simulink model "lunar_lander_sim_MPC"  (R2023a)
settings: Solver=VariableStepAuto  StartTime=0.0  StopTime=10.0  RelTol=1e-3
undefined symbols (not defined in the file or in its folder): A, aMode
libraries: simulink_extras x7, mpclib x2, shared6dofsys x2, sharedutil x2
settings Model: Creator=cnsl  LastModifiedBy=cnsl

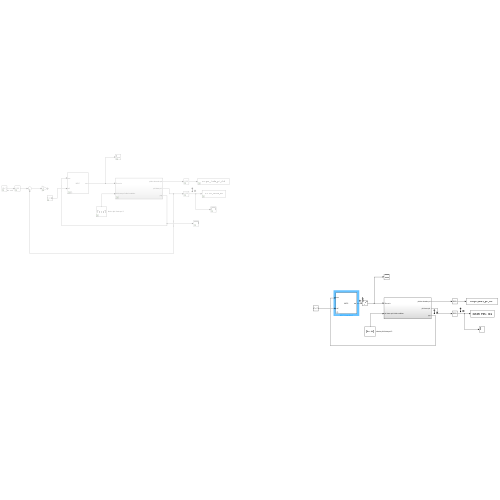
[thumbnail: Simulink's stored preview of the top-level diagram]
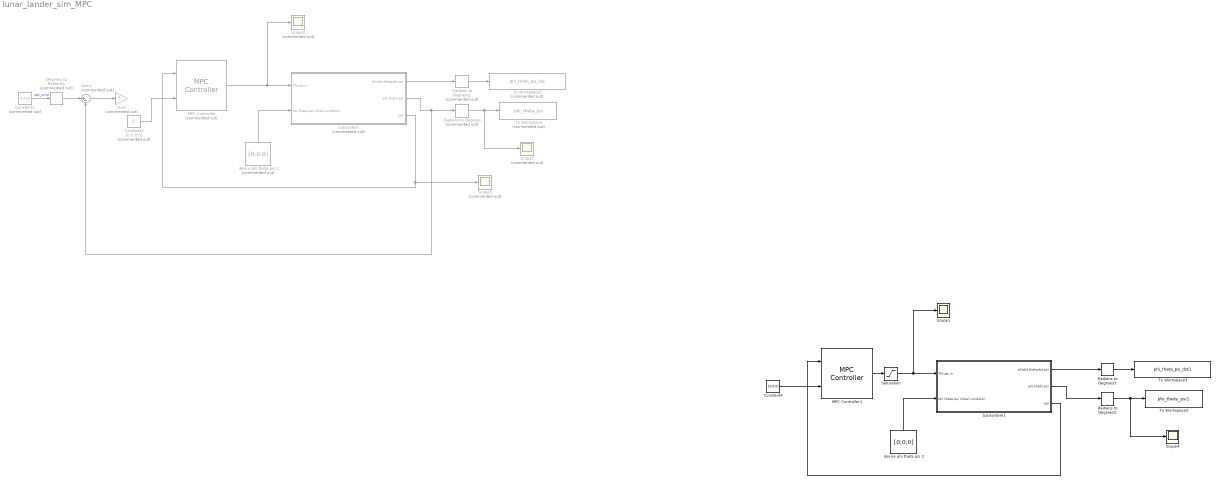
== system lunar_lander_sim_MPC ==
  Constant1 : Constant  Commented=on  Value=[5;0;0]
  Constant2 : Constant  Commented=on  Value=[0.5;0;0]
  Constant4 : Constant  Value=[0;0;0]
  Degrees to Radians1 : simulink_extras/Transformations/Degrees to Radians  Commented=on
  Gain : Gain  Commented=on  Gain=5
  MPC Controller : mpclib/MPC Controller  Commented=on  SCDEnableBlockLinearizationSpecification=on  mpcobj=mpc_stabilization_LL  is_multiple=0  enable_value=0  return_u0=off  updateMPCinCallerWorkspace=on  md_inport=off  mv_inport=off  uref_inport=off  return_cost=off  return_mvseq=off  return_qpstatus=off  return_xseq=off  return_state=off  return_ovseq=off  state_inport=off  umin_inport=off  umax_inport=off  ymin_inport=off  ymax_inport=off  cc_inport=off  ywt_inport=off  uwt_inport=off  duwt_inport=off  rhoeps_inport=off  pm_inport=off  MaximumP=10  HorizonChoice=FixedHorizon  n_ts=0.01  n_p=10  n_mv=8  n_md=0  n_ud=0  n_mo=3  n_uo=0  BlockDataType=double  SampleTimeInherited=off  switch_inport=off
  MPC Controller1 : mpclib/MPC Controller  SCDEnableBlockLinearizationSpecification=on  is_multiple=0  enable_value=0  return_u0=off  updateMPCinCallerWorkspace=on  md_inport=off  mv_inport=off  uref_inport=off  return_cost=off  return_mvseq=off  return_qpstatus=off  return_xseq=off  return_state=off  return_ovseq=off  state_inport=off  umin_inport=off  umax_inport=off  ymin_inport=off  ymax_inport=off  cc_inport=off  ywt_inport=off  uwt_inport=off  duwt_inport=off  rhoeps_inport=off  pm_inport=off  MaximumP=10  HorizonChoice=FixedHorizon  n_ts=0.1  n_p=10  n_mv=8  n_md=1  n_ud=0  n_mo=3  n_uo=0  BlockDataType=double  SampleTimeInherited=off  switch_inport=off
  Radians to Degrees : simulink_extras/Transformations/Radians to Degrees  Commented=on
  Radians to Degrees1 : simulink_extras/Transformations/Radians to Degrees  Commented=on
  Radians to Degrees2 : simulink_extras/Transformations/Radians to Degrees
  Radians to Degrees3 : simulink_extras/Transformations/Radians to Degrees
  Saturation : Saturate  UpperLimit=10  LowerLimit=0
  Scope1 : Scope
  Scope2 : Scope  Commented=on
  Scope3 : Scope  Commented=on
  Scope4 : Scope
  Scope5 : Scope  Commented=on
  Subsystem : Subsystem  Commented=on
  Subsystem1 : Subsystem
  Sum1 : Sum  Commented=on  Inputs=|+-
  To Workspace : ToWorkspace  Commented=on  VariableName=phi_theta_psi  SaveFormat=Timeseries  SampleTime=-1
  To Workspace1 : ToWorkspace  Commented=on  VariableName=phi_theta_psi_dot  SaveFormat=Timeseries  SampleTime=-1
  To Workspace2 : ToWorkspace  VariableName=phi_theta_psi1  SaveFormat=Timeseries  SampleTime=-1
  To Workspace3 : ToWorkspace  VariableName=phi_theta_psi_dot1  SaveFormat=Timeseries  SampleTime=-1
  desire phi theta psi 1 : Constant  Commented=on  Value=[0;0;0]
  desire phi theta psi 2 : Constant  Value=[0;0;0]
  wires:
  Subsystem/2("phi theta psi ") -> Radians to Degrees/1, Sum1/2
  Subsystem/1(phidot thetadot psi) -> Radians to Degrees1/1
  Radians to Degrees/1 -> Scope3/1, To Workspace/1
  desire phi theta psi 1/1 -> Subsystem/2("phi theta psi initial condition ")
  Radians to Degrees1/1 -> To Workspace1/1
  MPC Controller/1 -> Scope2/1, Subsystem/1(Thrust in)
  Subsystem/3(" pqr") -> Scope5/1, MPC Controller/1
  Constant1/1 -> Degrees to Radians1/1  "pqr_cmd"
  Degrees to Radians1/1 -> Sum1/1
  Sum1/1 -> Gain/1
  Constant2/1 -> MPC Controller/2
  Radians to Degrees2/1 -> Scope4/1, To Workspace2/1
  Subsystem1/2("phi theta psi ") -> Radians to Degrees2/1
  desire phi theta psi 2/1 -> Subsystem1/2("phi theta psi initial condition ")
  Radians to Degrees3/1 -> To Workspace3/1
  Constant4/1 -> MPC Controller1/2
  MPC Controller1/1 -> Saturation/1
  Subsystem1/1(phidot thetadot psi) -> Radians to Degrees3/1
  Subsystem1/3(" pqr") -> MPC Controller1/1
  Saturation/1 -> Scope1/1, Subsystem1/1(Thrust in)

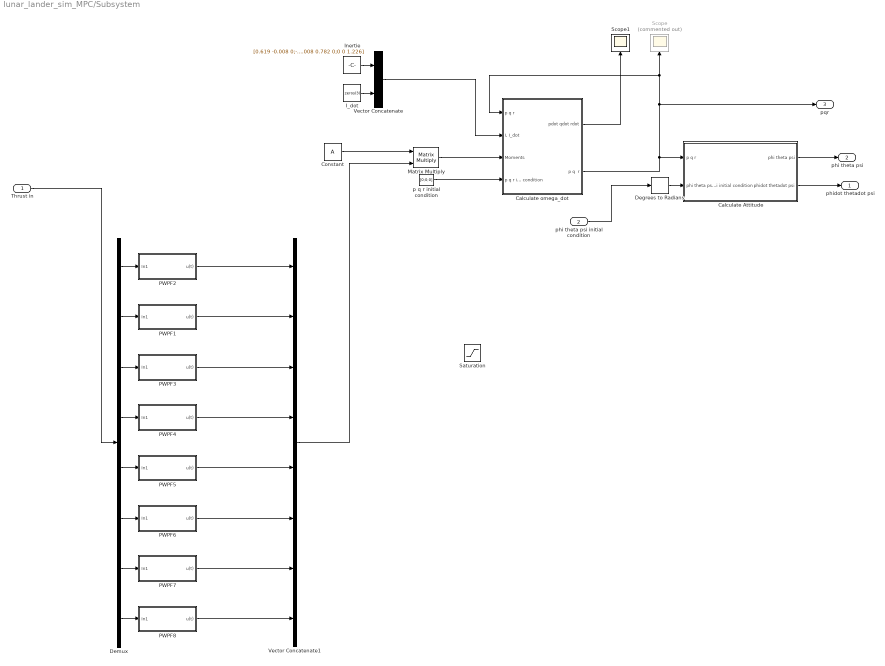
== system lunar_lander_sim_MPC/Subsystem ==
  Thrust in : Inport
  "phi theta psi initial condition " : Inport  Port=2
  " p q r initial condition" : Constant  Value=[0;0;0]
  "Calculate Attitude " : Subsystem
  Calculate omega_dot : Subsystem  AncestorBlock=shared6dofsys/Calculate omega_dot  mask{aMode=aMode}
      mask init:
      | if aerosharedtest(gcb)
      |     aerosharedicon('shared');
      | else
      |     sharedautoicon('shared');
      | end
      settings: LibrarySourceBlock=shared6dofsys/Calculate omega_dot
  Constant : Constant  Value=A
  Degrees to Radians : simulink_extras/Transformations/Degrees to Radians
  Demux : Demux  Outputs=8
  I_dot : Constant  Value=zeros(3)
  Inertie : Constant  Value=[0.619 -0.008 0;-0.008 0.782 0;0 0 1.226]
  Matrix Multiply : Product  Multiplication=Matrix(*)
  PWPF1 : Subsystem
  PWPF2 : Subsystem
  PWPF3 : Subsystem
  PWPF4 : Subsystem
  PWPF5 : Subsystem
  PWPF6 : Subsystem
  PWPF7 : Subsystem
  PWPF8 : Subsystem
  Saturation : Saturate
  Scope : Scope  Commented=on
  Scope1 : Scope
  Vector Concatenate : Concatenate  Mode=Multidimensional array
  Vector Concatenate1 : Concatenate  NumInputs=8
  phidot thetadot psi : Outport
  "phi theta psi " : Outport  Port=2
  " pqr" : Outport  Port=3
  wires:
  Vector Concatenate/1 -> Calculate omega_dot/2("I, I_dot")
  Inertie/1 -> Vector Concatenate/1
  Calculate omega_dot/2(p q  r) -> Scope/1, Calculate omega_dot/1(p q r), " pqr"/1, "Calculate Attitude "/1(p q r)
  I_dot/1 -> Vector Concatenate/2
  " p q r initial condition"/1 -> Calculate omega_dot/4(p q r initial condition)
  "Calculate Attitude "/1("phi theta psi ") -> "phi theta psi "/1
  Degrees to Radians/1 -> "Calculate Attitude "/2("phi theta psi initial condition ")
  "phi theta psi initial condition "/1 -> Degrees to Radians/1
  "Calculate Attitude "/2(phidot thetadot psi) -> phidot thetadot psi/1
  Calculate omega_dot/1(pdot qdot rdot) -> Scope1/1
  Matrix Multiply/1 -> Calculate omega_dot/3(Moments)
  Constant/1 -> Matrix Multiply/1
  Thrust in/1 -> Demux/1
  Demux/1 -> PWPF2/1(In1)
  Demux/2 -> PWPF1/1(In1)
  Demux/3 -> PWPF3/1(In1)
  Demux/4 -> PWPF4/1(In1)
  Demux/5 -> PWPF5/1(In1)
  Demux/6 -> PWPF6/1(In1)
  Demux/7 -> PWPF7/1(In1)
  Demux/8 -> PWPF8/1(In1)
  PWPF2/1(u(t)) -> Vector Concatenate1/1
  PWPF1/1(u(t)) -> Vector Concatenate1/2
  PWPF3/1(u(t)) -> Vector Concatenate1/3
  PWPF4/1(u(t)) -> Vector Concatenate1/4
  PWPF5/1(u(t)) -> Vector Concatenate1/5
  PWPF6/1(u(t)) -> Vector Concatenate1/6
  PWPF7/1(u(t)) -> Vector Concatenate1/7
  Vector Concatenate1/1 -> Matrix Multiply/2
  PWPF8/1(u(t)) -> Vector Concatenate1/8

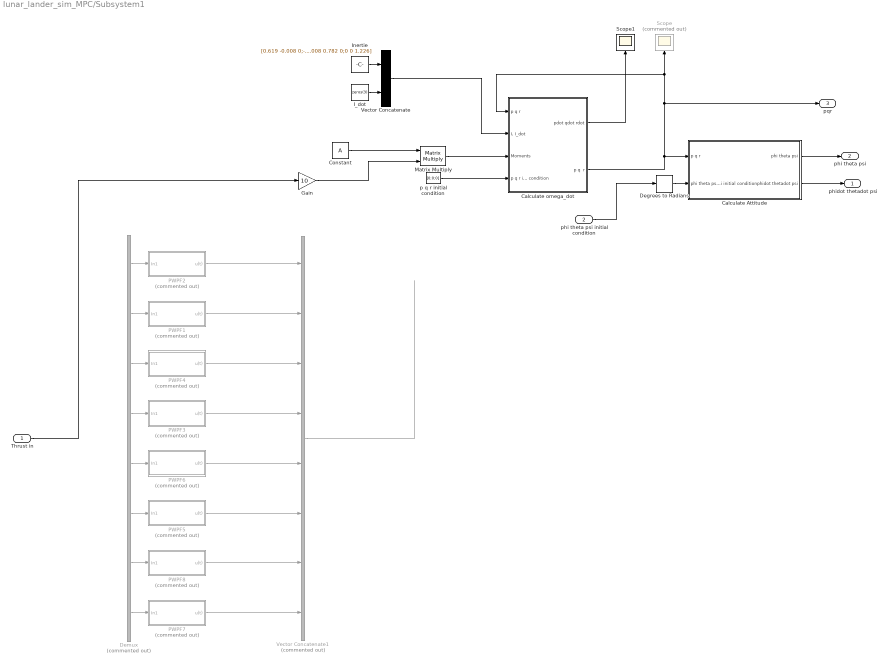
== system lunar_lander_sim_MPC/Subsystem1 ==
  Thrust in : Inport
  "phi theta psi initial condition " : Inport  Port=2
  " p q r initial condition" : Constant  Value=[0;0;0]
  "Calculate Attitude " : Subsystem
  Calculate omega_dot : Subsystem  AncestorBlock=shared6dofsys/Calculate omega_dot  mask{aMode=aMode}
      mask init:
      | if aerosharedtest(gcb)
      |     aerosharedicon('shared');
      | else
      |     sharedautoicon('shared');
      | end
      settings: LibrarySourceBlock=shared6dofsys/Calculate omega_dot
  Constant : Constant  Value=A
  Degrees to Radians : simulink_extras/Transformations/Degrees to Radians
  Demux : Demux  Commented=on  Outputs=8
  Gain : Gain  Gain=10
  I_dot : Constant  Value=zeros(3)
  Inertie : Constant  Value=[0.619 -0.008 0;-0.008 0.782 0;0 0 1.226]
  Matrix Multiply : Product  Multiplication=Matrix(*)
  PWPF1 : Subsystem  Commented=on
  PWPF2 : Subsystem  Commented=on
  PWPF3 : Subsystem  Commented=on
  PWPF4 : Subsystem  Commented=on
  PWPF5 : Subsystem  Commented=on
  PWPF6 : Subsystem  Commented=on
  PWPF7 : Subsystem  Commented=on
  PWPF8 : Subsystem  Commented=on
  Scope : Scope  Commented=on
  Scope1 : Scope
  Vector Concatenate : Concatenate  Mode=Multidimensional array
  Vector Concatenate1 : Concatenate  Commented=on  NumInputs=8
  phidot thetadot psi : Outport
  "phi theta psi " : Outport  Port=2
  " pqr" : Outport  Port=3
  wires:
  Vector Concatenate/1 -> Calculate omega_dot/2("I, I_dot")
  Inertie/1 -> Vector Concatenate/1
  Calculate omega_dot/2(p q  r) -> Scope/1, Calculate omega_dot/1(p q r), " pqr"/1, "Calculate Attitude "/1(p q r)
  I_dot/1 -> Vector Concatenate/2
  " p q r initial condition"/1 -> Calculate omega_dot/4(p q r initial condition)
  "Calculate Attitude "/1("phi theta psi ") -> "phi theta psi "/1
  Degrees to Radians/1 -> "Calculate Attitude "/2("phi theta psi initial condition ")
  "phi theta psi initial condition "/1 -> Degrees to Radians/1
  "Calculate Attitude "/2(phidot thetadot psi) -> phidot thetadot psi/1
  Calculate omega_dot/1(pdot qdot rdot) -> Scope1/1
  Matrix Multiply/1 -> Calculate omega_dot/3(Moments)
  Constant/1 -> Matrix Multiply/1
  Thrust in/1 -> Gain/1
  Demux/1 -> PWPF2/1(In1)
  Demux/2 -> PWPF1/1(In1)
  Demux/3 -> PWPF4/1(In1)
  Demux/4 -> PWPF3/1(In1)
  Demux/5 -> PWPF6/1(In1)
  Demux/6 -> PWPF5/1(In1)
  Demux/7 -> PWPF8/1(In1)
  Demux/8 -> PWPF7/1(In1)
  PWPF2/1(u(t)) -> Vector Concatenate1/1
  PWPF1/1(u(t)) -> Vector Concatenate1/2
  PWPF4/1(u(t)) -> Vector Concatenate1/3
  PWPF3/1(u(t)) -> Vector Concatenate1/4
  PWPF6/1(u(t)) -> Vector Concatenate1/5
  PWPF5/1(u(t)) -> Vector Concatenate1/6
  PWPF8/1(u(t)) -> Vector Concatenate1/7
  Vector Concatenate1/1 -> ?
  PWPF7/1(u(t)) -> Vector Concatenate1/8
  Gain/1 -> Matrix Multiply/2

== system lunar_lander_sim_MPC/Subsystem/Calculate Attitude  ==
  p q r : Inport
  "phi theta psi initial condition " : Inport  Port=2
  " " : Integrator  InitialConditionSource=external
  phidot thetadot psidot : shared6dofsys/DCM & Euler Angles (Euler)/phidot thetadot psidot  SystemSampleTime=-1  VariantActivationTime=update diagram  Latency=0  AutoFrameSizeCalculation=off
  "phi theta psi " : Outport
  phidot thetadot psi : Outport  Port=2
  wires:
  "phi theta psi initial condition "/1 -> " "/2
  " "/1 -> phidot thetadot psidot/2, "phi theta psi "/1
  phidot thetadot psidot/1 -> phidot thetadot psi/1, " "/1
  p q r/1 -> phidot thetadot psidot/1

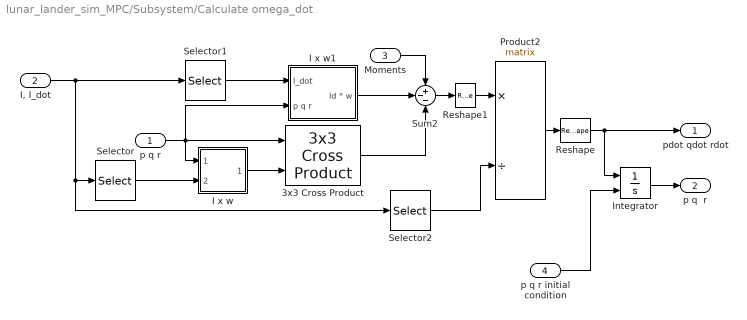
== system lunar_lander_sim_MPC/Subsystem/Calculate omega_dot ==
  p q r : Inport  OutDataTypeStr=double
  "I, I_dot" : Inport  Port=2  OutDataTypeStr=double
  Moments : Inport  Port=3  OutDataTypeStr=double
  p q r initial condition : Inport  Port=4
  3x3 Cross Product : sharedutil/3x3 Cross Product  aMode=aMode
  I x w : Subsystem
  I x w1 : Subsystem
  Integrator : Integrator  InitialConditionSource=external
  Product2 : Product  Inputs=*/  Multiplication=Matrix(*)  SaturateOnIntegerOverflow=on  OutDataTypeStr=Inherit: Same as first input
  Reshape : Reshape
  Reshape1 : Reshape  OutputDimensionality=Row vector (2-D)
  Selector : Selector  NumberOfDimensions=2  InputPortWidth=2  IndexOptions=Index vector (dialog),Select all  Indices=1:3,-1  OutputSizes=1
  Selector1 : Selector  NumberOfDimensions=2  InputPortWidth=2  IndexOptions=Index vector (dialog),Select all  Indices=4:6,-1  OutputSizes=1
  Selector2 : Selector  NumberOfDimensions=2  InputPortWidth=2  IndexOptions=Index vector (dialog),Select all  Indices=1:3,-1  OutputSizes=1
  Sum2 : Sum  Inputs=+--  SaturateOnIntegerOverflow=on
  pdot qdot rdot : Outport  OutDataTypeStr=double  VectorParamsAs1DForOutWhenUnconnected=off
  p q  r : Outport  Port=2
  wires:
  p q r initial condition/1 -> Integrator/2
  Integrator/1 -> p q  r/1
  Reshape/1 -> pdot qdot rdot/1, Integrator/1
  Selector/1 -> I x w/2(Inertia)
  Selector2/1 -> Product2/2
  "I, I_dot"/1 -> Selector/1, Selector2/1, Selector1/1
  p q r/1 -> 3x3 Cross Product/1, I x w1/2(p q r), I x w/1(p q r)
  Product2/1 -> Reshape/1
  Sum2/1 -> Reshape1/1
  Moments/1 -> Sum2/1
  I x w1/1(Id * w) -> Sum2/2
  Selector1/1 -> I x w1/1(I_dot)
  I x w/1(I * w) -> 3x3 Cross Product/2
  Reshape1/1 -> Product2/1
  3x3 Cross Product/1 -> Sum2/3

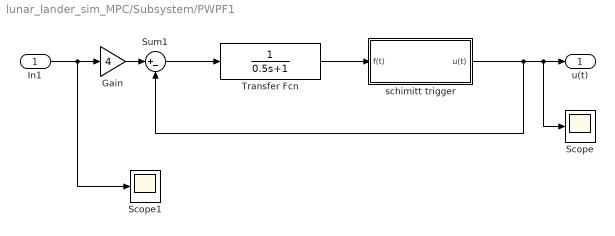
== system lunar_lander_sim_MPC/Subsystem/PWPF1 ==
  In1 : Inport
  Gain : Gain  Gain=4
  Scope : Scope
  Scope1 : Scope
  Sum1 : Sum  Inputs=|+-
  Transfer Fcn : TransferFcn  Denominator=[0.5 1]
  schimitt trigger : Subsystem
  u(t) : Outport
  wires:
  In1/1 -> Gain/1, Scope1/1
  Transfer Fcn/1 -> schimitt trigger/1(f(t))
  Sum1/1 -> Transfer Fcn/1
  Gain/1 -> Sum1/1
  schimitt trigger/1(u(t)) -> Sum1/2, u(t)/1, Scope/1

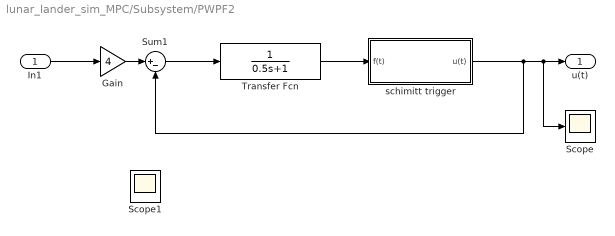
== system lunar_lander_sim_MPC/Subsystem/PWPF2 ==
  In1 : Inport
  Gain : Gain  Gain=4
  Scope : Scope
  Scope1 : Scope
  Sum1 : Sum  Inputs=|+-
  Transfer Fcn : TransferFcn  Denominator=[0.5 1]
  schimitt trigger : Subsystem
  u(t) : Outport
  wires:
  schimitt trigger/1(u(t)) -> Scope/1, u(t)/1, Sum1/2
  Gain/1 -> Sum1/1
  Sum1/1 -> Transfer Fcn/1
  Transfer Fcn/1 -> schimitt trigger/1(f(t))
  In1/1 -> Gain/1

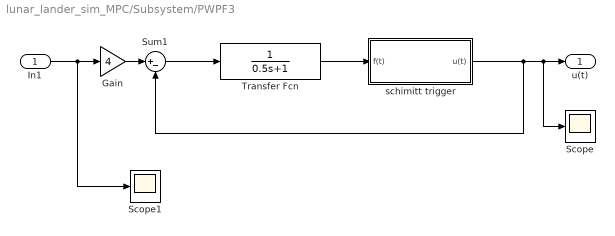
== system lunar_lander_sim_MPC/Subsystem/PWPF3 ==
  In1 : Inport
  Gain : Gain  Gain=4
  Scope : Scope
  Scope1 : Scope
  Sum1 : Sum  Inputs=|+-
  Transfer Fcn : TransferFcn  Denominator=[0.5 1]
  schimitt trigger : Subsystem
  u(t) : Outport
  wires:
  schimitt trigger/1(u(t)) -> Scope/1, u(t)/1, Sum1/2
  Gain/1 -> Sum1/1
  Sum1/1 -> Transfer Fcn/1
  Transfer Fcn/1 -> schimitt trigger/1(f(t))
  In1/1 -> Scope1/1, Gain/1

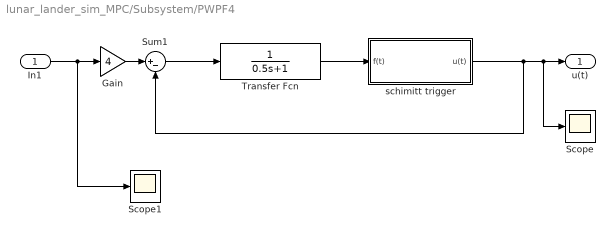
== system lunar_lander_sim_MPC/Subsystem/PWPF4 ==
  In1 : Inport
  Gain : Gain  Gain=4
  Scope : Scope
  Scope1 : Scope
  Sum1 : Sum  Inputs=|+-
  Transfer Fcn : TransferFcn  Denominator=[0.5 1]
  schimitt trigger : Subsystem
  u(t) : Outport
  wires:
  In1/1 -> Gain/1, Scope1/1
  Transfer Fcn/1 -> schimitt trigger/1(f(t))
  Sum1/1 -> Transfer Fcn/1
  Gain/1 -> Sum1/1
  schimitt trigger/1(u(t)) -> Sum1/2, u(t)/1, Scope/1

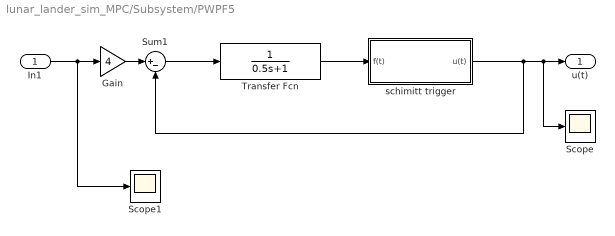
== system lunar_lander_sim_MPC/Subsystem/PWPF5 ==
  In1 : Inport
  Gain : Gain  Gain=4
  Scope : Scope
  Scope1 : Scope
  Sum1 : Sum  Inputs=|+-
  Transfer Fcn : TransferFcn  Denominator=[0.5 1]
  schimitt trigger : Subsystem
  u(t) : Outport
  wires:
  schimitt trigger/1(u(t)) -> Scope/1, u(t)/1, Sum1/2
  Gain/1 -> Sum1/1
  Sum1/1 -> Transfer Fcn/1
  Transfer Fcn/1 -> schimitt trigger/1(f(t))
  In1/1 -> Scope1/1, Gain/1

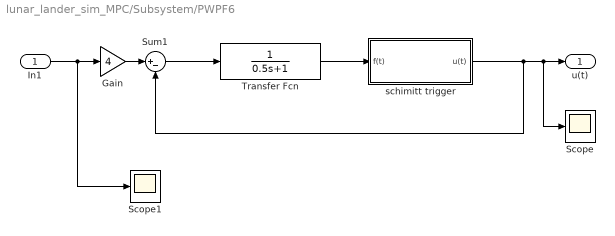
== system lunar_lander_sim_MPC/Subsystem/PWPF6 ==
  In1 : Inport
  Gain : Gain  Gain=4
  Scope : Scope
  Scope1 : Scope
  Sum1 : Sum  Inputs=|+-
  Transfer Fcn : TransferFcn  Denominator=[0.5 1]
  schimitt trigger : Subsystem
  u(t) : Outport
  wires:
  In1/1 -> Gain/1, Scope1/1
  Transfer Fcn/1 -> schimitt trigger/1(f(t))
  Sum1/1 -> Transfer Fcn/1
  Gain/1 -> Sum1/1
  schimitt trigger/1(u(t)) -> Sum1/2, u(t)/1, Scope/1

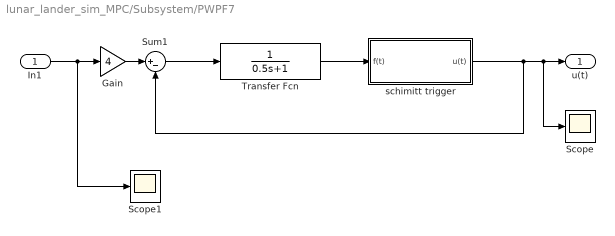
== system lunar_lander_sim_MPC/Subsystem/PWPF7 ==
  In1 : Inport
  Gain : Gain  Gain=4
  Scope : Scope
  Scope1 : Scope
  Sum1 : Sum  Inputs=|+-
  Transfer Fcn : TransferFcn  Denominator=[0.5 1]
  schimitt trigger : Subsystem
  u(t) : Outport
  wires:
  schimitt trigger/1(u(t)) -> Scope/1, u(t)/1, Sum1/2
  Gain/1 -> Sum1/1
  Sum1/1 -> Transfer Fcn/1
  Transfer Fcn/1 -> schimitt trigger/1(f(t))
  In1/1 -> Scope1/1, Gain/1

== system lunar_lander_sim_MPC/Subsystem/PWPF8 ==
  In1 : Inport
  Gain : Gain  Gain=4
  Scope : Scope
  Scope1 : Scope
  Sum1 : Sum  Inputs=|+-
  Transfer Fcn : TransferFcn  Denominator=[0.5 1]
  schimitt trigger : Subsystem
  u(t) : Outport
  wires:
  In1/1 -> Gain/1, Scope1/1
  Transfer Fcn/1 -> schimitt trigger/1(f(t))
  Sum1/1 -> Transfer Fcn/1
  Gain/1 -> Sum1/1
  schimitt trigger/1(u(t)) -> Sum1/2, u(t)/1, Scope/1

== system lunar_lander_sim_MPC/Subsystem1/Calculate Attitude  ==
  p q r : Inport
  "phi theta psi initial condition " : Inport  Port=2
  " " : Integrator  InitialConditionSource=external
  phidot thetadot psidot : shared6dofsys/DCM & Euler Angles (Euler)/phidot thetadot psidot  SystemSampleTime=-1  VariantActivationTime=update diagram  Latency=0  AutoFrameSizeCalculation=off
  "phi theta psi " : Outport
  phidot thetadot psi : Outport  Port=2
  wires:
  "phi theta psi initial condition "/1 -> " "/2
  " "/1 -> phidot thetadot psidot/2, "phi theta psi "/1
  phidot thetadot psidot/1 -> phidot thetadot psi/1, " "/1
  p q r/1 -> phidot thetadot psidot/1

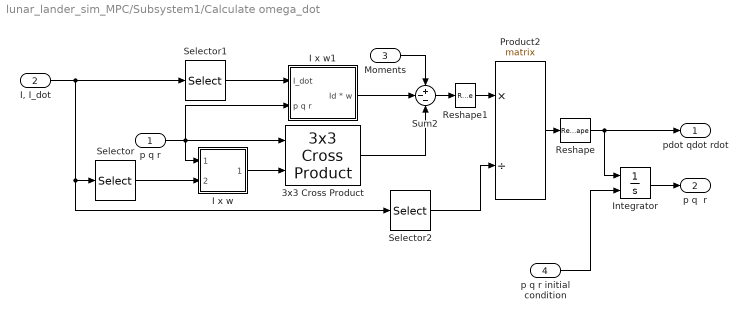
== system lunar_lander_sim_MPC/Subsystem1/Calculate omega_dot ==
  p q r : Inport  OutDataTypeStr=double
  "I, I_dot" : Inport  Port=2  OutDataTypeStr=double
  Moments : Inport  Port=3  OutDataTypeStr=double
  p q r initial condition : Inport  Port=4
  3x3 Cross Product : sharedutil/3x3 Cross Product  aMode=aMode
  I x w : Subsystem
  I x w1 : Subsystem
  Integrator : Integrator  InitialConditionSource=external
  Product2 : Product  Inputs=*/  Multiplication=Matrix(*)  SaturateOnIntegerOverflow=on  OutDataTypeStr=Inherit: Same as first input
  Reshape : Reshape
  Reshape1 : Reshape  OutputDimensionality=Row vector (2-D)
  Selector : Selector  NumberOfDimensions=2  InputPortWidth=2  IndexOptions=Index vector (dialog),Select all  Indices=1:3,-1  OutputSizes=1
  Selector1 : Selector  NumberOfDimensions=2  InputPortWidth=2  IndexOptions=Index vector (dialog),Select all  Indices=4:6,-1  OutputSizes=1
  Selector2 : Selector  NumberOfDimensions=2  InputPortWidth=2  IndexOptions=Index vector (dialog),Select all  Indices=1:3,-1  OutputSizes=1
  Sum2 : Sum  Inputs=+--  SaturateOnIntegerOverflow=on
  pdot qdot rdot : Outport  OutDataTypeStr=double  VectorParamsAs1DForOutWhenUnconnected=off
  p q  r : Outport  Port=2
  wires:
  p q r initial condition/1 -> Integrator/2
  Integrator/1 -> p q  r/1
  Reshape/1 -> pdot qdot rdot/1, Integrator/1
  Selector/1 -> I x w/2(Inertia)
  Selector2/1 -> Product2/2
  "I, I_dot"/1 -> Selector/1, Selector2/1, Selector1/1
  p q r/1 -> 3x3 Cross Product/1, I x w1/2(p q r), I x w/1(p q r)
  Product2/1 -> Reshape/1
  Sum2/1 -> Reshape1/1
  Moments/1 -> Sum2/1
  I x w1/1(Id * w) -> Sum2/2
  Selector1/1 -> I x w1/1(I_dot)
  I x w/1(I * w) -> 3x3 Cross Product/2
  Reshape1/1 -> Product2/1
  3x3 Cross Product/1 -> Sum2/3

== system lunar_lander_sim_MPC/Subsystem1/PWPF1 ==
  In1 : Inport
  Gain : Gain  Gain=4
  Scope : Scope
  Scope1 : Scope
  schimitt trigger : Subsystem
  u(t) : Outport
  wires:
  In1/1 -> Gain/1, Scope1/1
  Gain/1 -> schimitt trigger/1(f(t))
  schimitt trigger/1(u(t)) -> u(t)/1, Scope/1

== system lunar_lander_sim_MPC/Subsystem1/PWPF2 ==
  In1 : Inport
  Gain : Gain  Gain=4
  Scope : Scope
  Scope1 : Scope
  schimitt trigger : Subsystem
  u(t) : Outport
  wires:
  schimitt trigger/1(u(t)) -> Scope/1, u(t)/1
  Gain/1 -> schimitt trigger/1(f(t))
  In1/1 -> Scope1/1, Gain/1

== system lunar_lander_sim_MPC/Subsystem1/PWPF3 ==
  In1 : Inport
  Gain : Gain  Gain=4
  Scope : Scope
  Scope1 : Scope
  schimitt trigger : Subsystem
  u(t) : Outport
  wires:
  schimitt trigger/1(u(t)) -> Scope/1, u(t)/1
  Gain/1 -> schimitt trigger/1(f(t))
  In1/1 -> Scope1/1, Gain/1

== system lunar_lander_sim_MPC/Subsystem1/PWPF4 ==
  In1 : Inport
  Gain : Gain  Gain=4
  Scope : Scope
  Scope1 : Scope
  schimitt trigger : Subsystem
  u(t) : Outport
  wires:
  In1/1 -> Gain/1, Scope1/1
  Gain/1 -> schimitt trigger/1(f(t))
  schimitt trigger/1(u(t)) -> u(t)/1, Scope/1

== system lunar_lander_sim_MPC/Subsystem1/PWPF5 ==
  In1 : Inport
  Gain : Gain  Gain=4
  Scope : Scope
  Scope1 : Scope
  schimitt trigger : Subsystem
  u(t) : Outport
  wires:
  schimitt trigger/1(u(t)) -> Scope/1, u(t)/1
  Gain/1 -> schimitt trigger/1(f(t))
  In1/1 -> Scope1/1, Gain/1

== system lunar_lander_sim_MPC/Subsystem1/PWPF6 ==
  In1 : Inport
  Gain : Gain  Gain=4
  Scope : Scope
  Scope1 : Scope
  schimitt trigger : Subsystem
  u(t) : Outport
  wires:
  In1/1 -> Gain/1, Scope1/1
  Gain/1 -> schimitt trigger/1(f(t))
  schimitt trigger/1(u(t)) -> u(t)/1, Scope/1

== system lunar_lander_sim_MPC/Subsystem1/PWPF7 ==
  In1 : Inport
  Gain : Gain  Gain=4
  Scope : Scope
  Scope1 : Scope
  schimitt trigger : Subsystem
  u(t) : Outport
  wires:
  In1/1 -> Gain/1, Scope1/1
  Gain/1 -> schimitt trigger/1(f(t))
  schimitt trigger/1(u(t)) -> u(t)/1, Scope/1

== system lunar_lander_sim_MPC/Subsystem1/PWPF8 ==
  In1 : Inport
  Gain : Gain  Gain=4
  Scope : Scope
  Scope1 : Scope
  schimitt trigger : Subsystem
  u(t) : Outport
  wires:
  schimitt trigger/1(u(t)) -> Scope/1, u(t)/1
  Gain/1 -> schimitt trigger/1(f(t))
  In1/1 -> Scope1/1, Gain/1

== system lunar_lander_sim_MPC/Subsystem/Calculate omega_dot/I x w ==
  p q r : Inport
  Inertia : Inport  Port=2
  Product : Product  Multiplication=Matrix(*)  InputSameDT=on  SaturateOnIntegerOverflow=on  OutDataTypeStr=Inherit: Same as first input
  Reshape1 : Reshape  OutputDimensionality=Column vector (2-D)
  Reshape2 : Reshape
  I * w : Outport  VectorParamsAs1DForOutWhenUnconnected=off
  wires:
  Product/1 -> Reshape2/1
  Inertia/1 -> Product/1
  p q r/1 -> Reshape1/1
  Reshape1/1 -> Product/2
  Reshape2/1 -> I * w/1

== system lunar_lander_sim_MPC/Subsystem/Calculate omega_dot/I x w1 ==
  I_dot : Inport
  p q r : Inport  Port=2
  Product : Product  Multiplication=Matrix(*)  InputSameDT=on  SaturateOnIntegerOverflow=on  OutDataTypeStr=Inherit: Same as first input
  Reshape1 : Reshape  OutputDimensionality=Column vector (2-D)
  Reshape2 : Reshape
  Id * w : Outport  VectorParamsAs1DForOutWhenUnconnected=off
  wires:
  p q r/1 -> Reshape1/1
  I_dot/1 -> Product/1
  Product/1 -> Reshape2/1
  Reshape1/1 -> Product/2
  Reshape2/1 -> Id * w/1

== system lunar_lander_sim_MPC/Subsystem/PWPF1/schimitt trigger ==
  f(t) : Inport
  Gain : Gain  Gain=-1
  Relay : Relay  OnSwitchValue=0.45  OffSwitchValue=0.15  OnOutputValue=10
  Relay1 : Relay  OnSwitchValue=0.45  OffSwitchValue=0.15  OnOutputValue=-10
  Switch : Switch  Criteria=u2 > Threshold  SaturateOnIntegerOverflow=off  InputSameDT=off
  u(t) : Outport
  wires:
  Switch/1 -> u(t)/1
  Relay/1 -> Switch/1
  Gain/1 -> Relay1/1
  Relay1/1 -> Switch/3
  f(t)/1 -> Switch/2, Gain/1, Relay/1

== system lunar_lander_sim_MPC/Subsystem/PWPF2/schimitt trigger ==
  f(t) : Inport
  Gain : Gain  Gain=-1
  Relay : Relay  OnSwitchValue=0.45  OffSwitchValue=0.15  OnOutputValue=10
  Relay1 : Relay  OnSwitchValue=0.45  OffSwitchValue=0.15  OnOutputValue=-10
  Switch : Switch  Criteria=u2 > Threshold  SaturateOnIntegerOverflow=off  InputSameDT=off
  u(t) : Outport
  wires:
  f(t)/1 -> Relay/1, Gain/1, Switch/2
  Relay1/1 -> Switch/3
  Gain/1 -> Relay1/1
  Relay/1 -> Switch/1
  Switch/1 -> u(t)/1

== system lunar_lander_sim_MPC/Subsystem/PWPF3/schimitt trigger ==
  f(t) : Inport
  Gain : Gain  Gain=-1
  Relay : Relay  OnSwitchValue=0.45  OffSwitchValue=0.15  OnOutputValue=10
  Relay1 : Relay  OnSwitchValue=0.45  OffSwitchValue=0.15  OnOutputValue=-10
  Switch : Switch  Criteria=u2 > Threshold  SaturateOnIntegerOverflow=off  InputSameDT=off
  u(t) : Outport
  wires:
  f(t)/1 -> Relay/1, Gain/1, Switch/2
  Relay1/1 -> Switch/3
  Gain/1 -> Relay1/1
  Relay/1 -> Switch/1
  Switch/1 -> u(t)/1

== system lunar_lander_sim_MPC/Subsystem/PWPF4/schimitt trigger ==
  f(t) : Inport
  Gain : Gain  Gain=-1
  Relay : Relay  OnSwitchValue=0.45  OffSwitchValue=0.15  OnOutputValue=10
  Relay1 : Relay  OnSwitchValue=0.45  OffSwitchValue=0.15  OnOutputValue=-10
  Switch : Switch  Criteria=u2 > Threshold  SaturateOnIntegerOverflow=off  InputSameDT=off
  u(t) : Outport
  wires:
  Switch/1 -> u(t)/1
  Relay/1 -> Switch/1
  Gain/1 -> Relay1/1
  Relay1/1 -> Switch/3
  f(t)/1 -> Switch/2, Gain/1, Relay/1

== system lunar_lander_sim_MPC/Subsystem/PWPF5/schimitt trigger ==
  f(t) : Inport
  Gain : Gain  Gain=-1
  Relay : Relay  OnSwitchValue=0.45  OffSwitchValue=0.15  OnOutputValue=10
  Relay1 : Relay  OnSwitchValue=0.45  OffSwitchValue=0.15  OnOutputValue=-10
  Switch : Switch  Criteria=u2 > Threshold  SaturateOnIntegerOverflow=off  InputSameDT=off
  u(t) : Outport
  wires:
  f(t)/1 -> Relay/1, Gain/1, Switch/2
  Relay1/1 -> Switch/3
  Gain/1 -> Relay1/1
  Relay/1 -> Switch/1
  Switch/1 -> u(t)/1

== system lunar_lander_sim_MPC/Subsystem/PWPF6/schimitt trigger ==
  f(t) : Inport
  Gain : Gain  Gain=-1
  Relay : Relay  OnSwitchValue=0.45  OffSwitchValue=0.15  OnOutputValue=10
  Relay1 : Relay  OnSwitchValue=0.45  OffSwitchValue=0.15  OnOutputValue=-10
  Switch : Switch  Criteria=u2 > Threshold  SaturateOnIntegerOverflow=off  InputSameDT=off
  u(t) : Outport
  wires:
  Switch/1 -> u(t)/1
  Relay/1 -> Switch/1
  Gain/1 -> Relay1/1
  Relay1/1 -> Switch/3
  f(t)/1 -> Switch/2, Gain/1, Relay/1

== system lunar_lander_sim_MPC/Subsystem/PWPF7/schimitt trigger ==
  f(t) : Inport
  Gain : Gain  Gain=-1
  Relay : Relay  OnSwitchValue=0.45  OffSwitchValue=0.15  OnOutputValue=10
  Relay1 : Relay  OnSwitchValue=0.45  OffSwitchValue=0.15  OnOutputValue=-10
  Switch : Switch  Criteria=u2 > Threshold  SaturateOnIntegerOverflow=off  InputSameDT=off
  u(t) : Outport
  wires:
  f(t)/1 -> Relay/1, Gain/1, Switch/2
  Relay1/1 -> Switch/3
  Gain/1 -> Relay1/1
  Relay/1 -> Switch/1
  Switch/1 -> u(t)/1

== system lunar_lander_sim_MPC/Subsystem/PWPF8/schimitt trigger ==
  f(t) : Inport
  Gain : Gain  Gain=-1
  Relay : Relay  OnSwitchValue=0.45  OffSwitchValue=0.15  OnOutputValue=10
  Relay1 : Relay  OnSwitchValue=0.45  OffSwitchValue=0.15  OnOutputValue=-10
  Switch : Switch  Criteria=u2 > Threshold  SaturateOnIntegerOverflow=off  InputSameDT=off
  u(t) : Outport
  wires:
  Switch/1 -> u(t)/1
  Relay/1 -> Switch/1
  Gain/1 -> Relay1/1
  Relay1/1 -> Switch/3
  f(t)/1 -> Switch/2, Gain/1, Relay/1

== system lunar_lander_sim_MPC/Subsystem1/Calculate omega_dot/I x w ==
  p q r : Inport
  Inertia : Inport  Port=2
  Product : Product  Multiplication=Matrix(*)  InputSameDT=on  SaturateOnIntegerOverflow=on  OutDataTypeStr=Inherit: Same as first input
  Reshape1 : Reshape  OutputDimensionality=Column vector (2-D)
  Reshape2 : Reshape
  I * w : Outport  VectorParamsAs1DForOutWhenUnconnected=off
  wires:
  Product/1 -> Reshape2/1
  Inertia/1 -> Product/1
  p q r/1 -> Reshape1/1
  Reshape1/1 -> Product/2
  Reshape2/1 -> I * w/1

== system lunar_lander_sim_MPC/Subsystem1/Calculate omega_dot/I x w1 ==
  I_dot : Inport
  p q r : Inport  Port=2
  Product : Product  Multiplication=Matrix(*)  InputSameDT=on  SaturateOnIntegerOverflow=on  OutDataTypeStr=Inherit: Same as first input
  Reshape1 : Reshape  OutputDimensionality=Column vector (2-D)
  Reshape2 : Reshape
  Id * w : Outport  VectorParamsAs1DForOutWhenUnconnected=off
  wires:
  p q r/1 -> Reshape1/1
  I_dot/1 -> Product/1
  Product/1 -> Reshape2/1
  Reshape1/1 -> Product/2
  Reshape2/1 -> Id * w/1

== system lunar_lander_sim_MPC/Subsystem1/PWPF1/schimitt trigger ==
  f(t) : Inport
  Relay : Relay  OnSwitchValue=0.45  OffSwitchValue=0.15  OnOutputValue=10
  u(t) : Outport
  wires:
  Relay/1 -> u(t)/1
  f(t)/1 -> Relay/1

== system lunar_lander_sim_MPC/Subsystem1/PWPF2/schimitt trigger ==
  f(t) : Inport
  Relay : Relay  OnSwitchValue=0.45  OffSwitchValue=0.15  OnOutputValue=10
  u(t) : Outport
  wires:
  f(t)/1 -> Relay/1
  Relay/1 -> u(t)/1

== system lunar_lander_sim_MPC/Subsystem1/PWPF3/schimitt trigger ==
  f(t) : Inport
  Relay : Relay  OnSwitchValue=0.45  OffSwitchValue=0.15  OnOutputValue=10
  u(t) : Outport
  wires:
  f(t)/1 -> Relay/1
  Relay/1 -> u(t)/1

== system lunar_lander_sim_MPC/Subsystem1/PWPF4/schimitt trigger ==
  f(t) : Inport
  Relay : Relay  OnSwitchValue=0.45  OffSwitchValue=0.15  OnOutputValue=10
  u(t) : Outport
  wires:
  Relay/1 -> u(t)/1
  f(t)/1 -> Relay/1

== system lunar_lander_sim_MPC/Subsystem1/PWPF5/schimitt trigger ==
  f(t) : Inport
  Relay : Relay  OnSwitchValue=0.45  OffSwitchValue=0.15  OnOutputValue=10
  u(t) : Outport
  wires:
  f(t)/1 -> Relay/1
  Relay/1 -> u(t)/1

== system lunar_lander_sim_MPC/Subsystem1/PWPF6/schimitt trigger ==
  f(t) : Inport
  Relay : Relay  OnSwitchValue=0.45  OffSwitchValue=0.15  OnOutputValue=10
  u(t) : Outport
  wires:
  Relay/1 -> u(t)/1
  f(t)/1 -> Relay/1

== system lunar_lander_sim_MPC/Subsystem1/PWPF7/schimitt trigger ==
  f(t) : Inport
  Relay : Relay  OnSwitchValue=0.45  OffSwitchValue=0.15  OnOutputValue=10
  u(t) : Outport
  wires:
  Relay/1 -> u(t)/1
  f(t)/1 -> Relay/1

== system lunar_lander_sim_MPC/Subsystem1/PWPF8/schimitt trigger ==
  f(t) : Inport
  Relay : Relay  OnSwitchValue=0.45  OffSwitchValue=0.15  OnOutputValue=10
  u(t) : Outport
  wires:
  f(t)/1 -> Relay/1
  Relay/1 -> u(t)/1
